simulink subsystem "rss_ChipFaltDia"  (R2023a)
settings: Solver=VariableStepAuto  StartTime=0.0  StopTime=10.0  RelTol=1e-3
undefined symbols (not defined in the file): ENM_TYPE_FALT, Gu16_ctChipFaltConfCnt_C, Gu16_ctChipFaltRcvyCnt_C
libraries: lib_debounce x1, lib_fault_definiteness x1
settings Model: Creator=xiaoqiang.yuan  LastModifiedBy=yunqi.lu

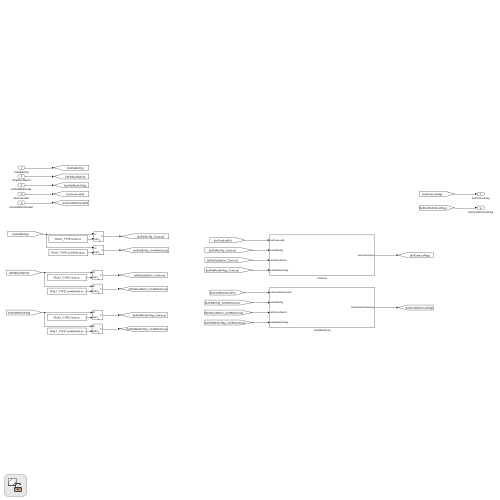
[thumbnail: Simulink's stored preview of the top-level diagram]
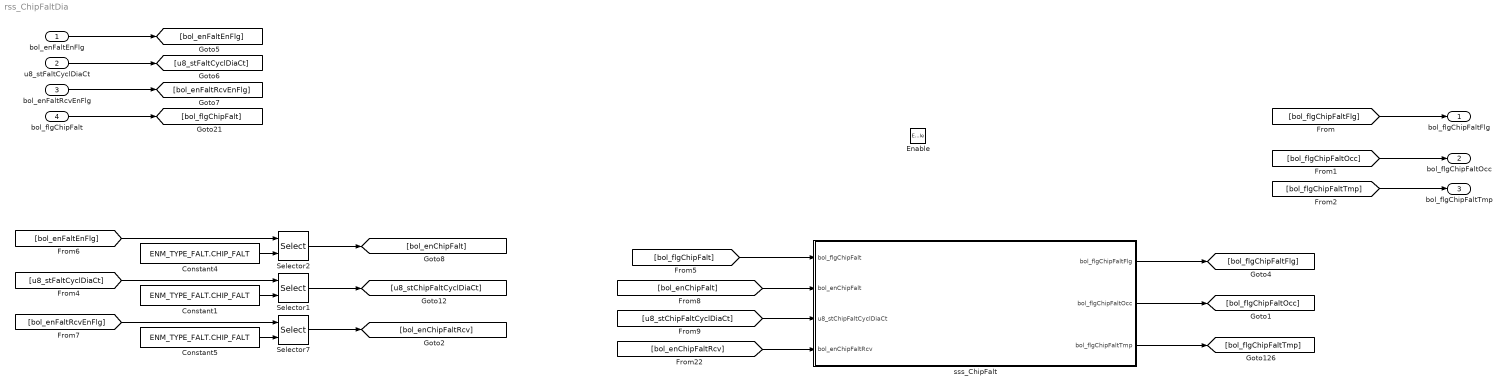
== system rss_ChipFaltDia ==
  bol_enFaltEnFlg : Inport  OutDataTypeStr=boolean
  u8_stFaltCyclDiaCt : Inport  Port=2  OutDataTypeStr=uint8
  bol_enFaltRcvEnFlg : Inport  Port=3  OutDataTypeStr=boolean
  bol_flgChipFalt : Inport  Port=4  OutDataTypeStr=boolean
  Enable : EnablePort
  Constant1 : Constant  Value=ENM_TYPE_FALT.CHIP_FALT
  Constant4 : Constant  Value=ENM_TYPE_FALT.CHIP_FALT
  Constant5 : Constant  Value=ENM_TYPE_FALT.CHIP_FALT
  Selector1 : Selector  IndexMode=Zero-based  InputPortWidth=Cdbl_numFaltDiaNum  IndexOptions=Index vector (port)  Indices=[1 3]  OutputSizes=1
  Selector2 : Selector  IndexMode=Zero-based  InputPortWidth=Cdbl_numFaltDiaNum  IndexOptions=Index vector (port)  Indices=[1 3]  OutputSizes=1
  Selector7 : Selector  IndexMode=Zero-based  InputPortWidth=Cdbl_numFaltDiaNum  IndexOptions=Index vector (port)  Indices=[1 3]  OutputSizes=1
  sss_ChipFalt : Subsystem
  bol_flgChipFaltFlg : Outport  OutDataTypeStr=boolean
  bol_flgChipFaltOcc : Outport  Port=2  OutDataTypeStr=boolean
  bol_flgChipFaltTmp : Outport  Port=3  OutDataTypeStr=boolean
  wires:
  [bol_flgChipFaltFlg] -> bol_flgChipFaltFlg/1
  [u8_stFaltCyclDiaCt] -> Selector1/1
  [bol_enFaltEnFlg] -> Selector2/1
  bol_enFaltEnFlg/1 -> [bol_enFaltEnFlg]
  bol_enFaltRcvEnFlg/1 -> [bol_enFaltRcvEnFlg]
  [bol_flgChipFalt] -> sss_ChipFalt/1(bol_flgChipFalt)
  Constant1/1 -> Selector1/2
  [u8_stChipFaltCyclDiaCt] -> sss_ChipFalt/3(u8_stChipFaltCyclDiaCt)
  [bol_enChipFalt] -> sss_ChipFalt/2(bol_enChipFalt)
  Constant4/1 -> Selector2/2
  Constant5/1 -> Selector7/2
  Selector1/1 -> [u8_stChipFaltCyclDiaCt]
  bol_flgChipFalt/1 -> [bol_flgChipFalt]
  Selector7/1 -> [bol_enChipFaltRcv]
  [bol_enFaltRcvEnFlg] -> Selector7/1
  Selector2/1 -> [bol_enChipFalt]
  [bol_enChipFaltRcv] -> sss_ChipFalt/4(bol_enChipFaltRcv)
  u8_stFaltCyclDiaCt/1 -> [u8_stFaltCyclDiaCt]
  sss_ChipFalt/1(bol_flgChipFaltFlg) -> [bol_flgChipFaltFlg]
  sss_ChipFalt/2(bol_flgChipFaltOcc) -> [bol_flgChipFaltOcc]
  [bol_flgChipFaltOcc] -> bol_flgChipFaltOcc/1
  [bol_flgChipFaltTmp] -> bol_flgChipFaltTmp/1
  sss_ChipFalt/3(bol_flgChipFaltTmp) -> [bol_flgChipFaltTmp]

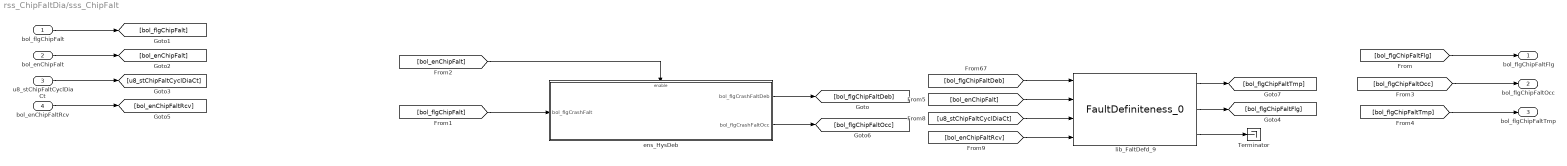
== system rss_ChipFaltDia/sss_ChipFalt ==
  bol_flgChipFalt : Inport
  bol_enChipFalt : Inport  Port=2
  u8_stChipFaltCyclDiaCt : Inport  Port=3
  bol_enChipFaltRcv : Inport  Port=4
  Terminator : Terminator
  ens_HysDeb : Subsystem
  lib_FaltDefd_9 : lib_fault_definiteness/FaultDefiniteness_0  lb_FaltWaitRecvCnt=Gu16_ctChipFaltConfCnt_C
  bol_flgChipFaltFlg : Outport
  bol_flgChipFaltOcc : Outport  Port=2
  bol_flgChipFaltTmp : Outport  Port=3
  wires:
  [bol_flgChipFaltTmp] -> bol_flgChipFaltTmp/1
  [bol_flgChipFaltOcc] -> bol_flgChipFaltOcc/1
  ens_HysDeb/2(bol_flgCrashFaltOcc) -> [bol_flgChipFaltOcc]
  lib_FaltDefd_9/1 -> [bol_flgChipFaltTmp]
  lib_FaltDefd_9/2 -> [bol_flgChipFaltFlg]
  lib_FaltDefd_9/3 -> Terminator/1
  [bol_enChipFalt] -> ens_HysDeb/Enable
  [bol_flgChipFalt] -> ens_HysDeb/1(bol_flgCrashFalt)
  ens_HysDeb/1(bol_flgCrashFaltDeb) -> [bol_flgChipFaltDeb]
  bol_enChipFaltRcv/1 -> [bol_enChipFaltRcv]
  u8_stChipFaltCyclDiaCt/1 -> [u8_stChipFaltCyclDiaCt]
  bol_enChipFalt/1 -> [bol_enChipFalt]
  [bol_flgChipFaltFlg] -> bol_flgChipFaltFlg/1
  bol_flgChipFalt/1 -> [bol_flgChipFalt]
  [bol_enChipFaltRcv] -> lib_FaltDefd_9/4
  [u8_stChipFaltCyclDiaCt] -> lib_FaltDefd_9/3
  [bol_enChipFalt] -> lib_FaltDefd_9/2
  [bol_flgChipFaltDeb] -> lib_FaltDefd_9/1

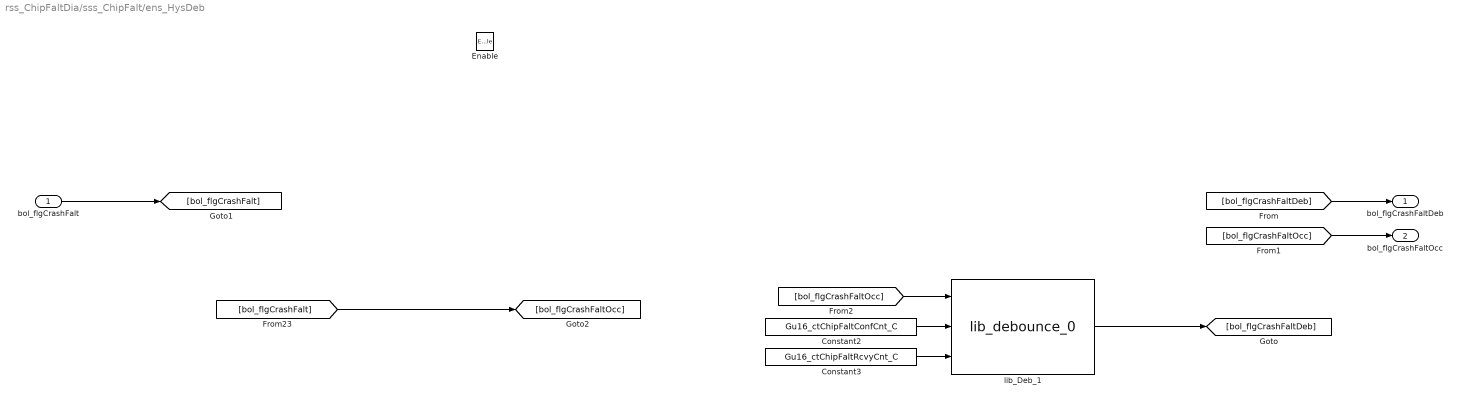
== system rss_ChipFaltDia/sss_ChipFalt/ens_HysDeb ==
  bol_flgCrashFalt : Inport
  Enable : EnablePort
  Constant2 : Constant  Value=Gu16_ctChipFaltConfCnt_C
  Constant3 : Constant  Value=Gu16_ctChipFaltRcvyCnt_C
  lib_Deb_1 : lib_debounce/lib_debounce_0
  bol_flgCrashFaltDeb : Outport
  bol_flgCrashFaltOcc : Outport  Port=2
  wires:
  [bol_flgCrashFaltOcc] -> lib_Deb_1/1
  [bol_flgCrashFalt] -> [bol_flgCrashFaltOcc]
  [bol_flgCrashFaltOcc] -> bol_flgCrashFaltOcc/1
  lib_Deb_1/1 -> [bol_flgCrashFaltDeb]
  bol_flgCrashFalt/1 -> [bol_flgCrashFalt]
  [bol_flgCrashFaltDeb] -> bol_flgCrashFaltDeb/1
  Constant3/1 -> lib_Deb_1/3
  Constant2/1 -> lib_Deb_1/2
